simulink model "Gesamtmodell_Bahnplanung"  (R2015b)
settings: Solver=ode3  StartTime=0.0  StopTime=inf  FixedStep=dt  RelTol=1e-3
InitFcn:
  | Reglerauslegung
undefined symbols (not defined in the file): aMax, aMaxPsi, Blindzeit, Com1, dt, K1, K2, K3, Kx, Ky, none, sigbuilder_block, Tx, Ty, vMax, vMaxPsi
libraries: xpcrtudplib x11, simulink x6, xpcutilitieslib x4, xpcseriallib x1, slrtlib x1
(part 2 of 4)

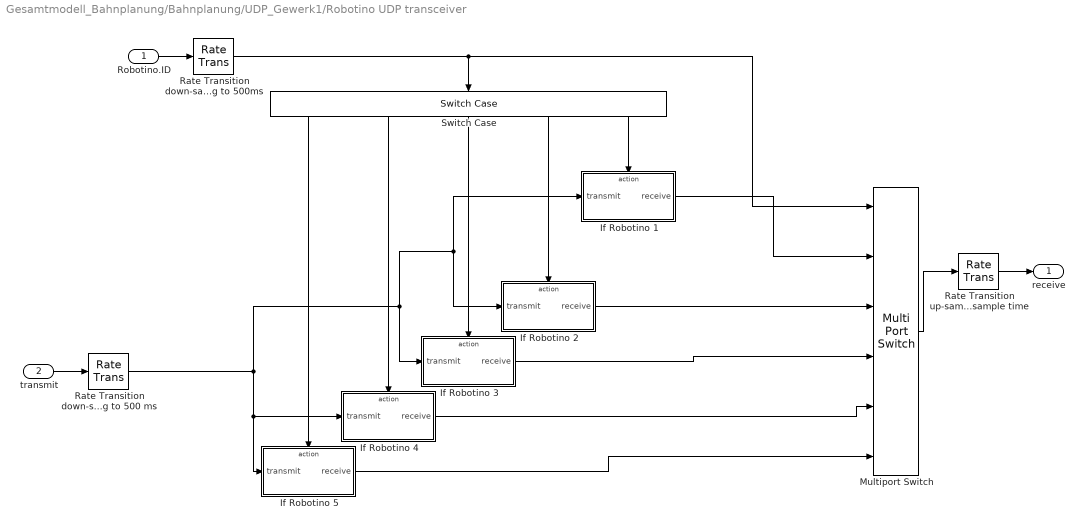
== system Gesamtmodell_Bahnplanung/Bahnplanung/UDP_Gewerk1/Robotino UDP transceiver ==
  Robotino.ID : Inport
  transmit : Inport  Port=2
  If Robotino 1 : Subsystem  TreatAsAtomicUnit=on
  If Robotino 2 : Subsystem  TreatAsAtomicUnit=on
  If Robotino 3 : Subsystem  TreatAsAtomicUnit=on
  If Robotino 4 : Subsystem  TreatAsAtomicUnit=on
  If Robotino 5 : Subsystem  TreatAsAtomicUnit=on
  Multiport Switch : MultiPortSwitch  Inputs=5
  Rate Transition down-sampling to 500 ms : RateTransition  OutPortSampleTime=0.5
  Rate Transition down-sampling to 500ms : RateTransition  OutPortSampleTime=0.5
  Rate Transition up-sampling to fundamental sample time : RateTransition
  Switch Case : SwitchCase  CaseConditions={5,4,3,2,1}  ShowDefaultCase=off
  receive : Outport
  wires:
  If Robotino 5/1(receive) -> Multiport Switch/6
  Switch Case/1 -> If Robotino 5/Action
  Rate Transition down-sampling to 500ms/1 -> Multiport Switch/1, Switch Case/1
  Robotino.ID/1 -> Rate Transition down-sampling to 500ms/1
  Rate Transition down-sampling to 500 ms/1 -> If Robotino 4/1(transmit), If Robotino 5/1(transmit), If Robotino 1/1(transmit), If Robotino 2/1(transmit), If Robotino 3/1(transmit)
  Rate Transition up-sampling to fundamental sample time/1 -> receive/1
  transmit/1 -> Rate Transition down-sampling to 500 ms/1
  If Robotino 4/1(receive) -> Multiport Switch/5
  If Robotino 2/1(receive) -> Multiport Switch/3
  If Robotino 3/1(receive) -> Multiport Switch/4
  If Robotino 1/1(receive) -> Multiport Switch/2
  Multiport Switch/1 -> Rate Transition up-sampling to fundamental sample time/1
  Switch Case/5 -> If Robotino 1/Action
  Switch Case/4 -> If Robotino 2/Action
  Switch Case/3 -> If Robotino 3/Action
  Switch Case/2 -> If Robotino 4/Action

== system Gesamtmodell_Bahnplanung/Regelung1/Receiver/UDP interface ==
  number of robot : Inport
  Receive : xpcrtudplib/UDP Receive  ipAddressVal=Use host-target connection  localPort=25000  rcvWidth=448  rcvFmAny=off  fmAddress=0.0.0.0  maxUDPQueue=8  sampleTime=-1
  Terminator : Terminator
  Unpack : xpcutilitieslib/Byte Unpacking   MaskUnpackedDataTypes={'double'}  MaskUnpackedDataSizes={[56]}  MaskAlignment=1
  stop signals : MATLAB Function  TreatAsAtomicUnit=on
  enable : Outport
  UDP data : Outport  Port=2
  wires:
  Unpack/1 -> stop signals/2(udp_in), UDP data/1
  Receive/1 -> Unpack/1
  Receive/2 -> Terminator/1
  stop signals/1(enable_out) -> enable/1
  number of robot/1 -> stop signals/1(rob_number)

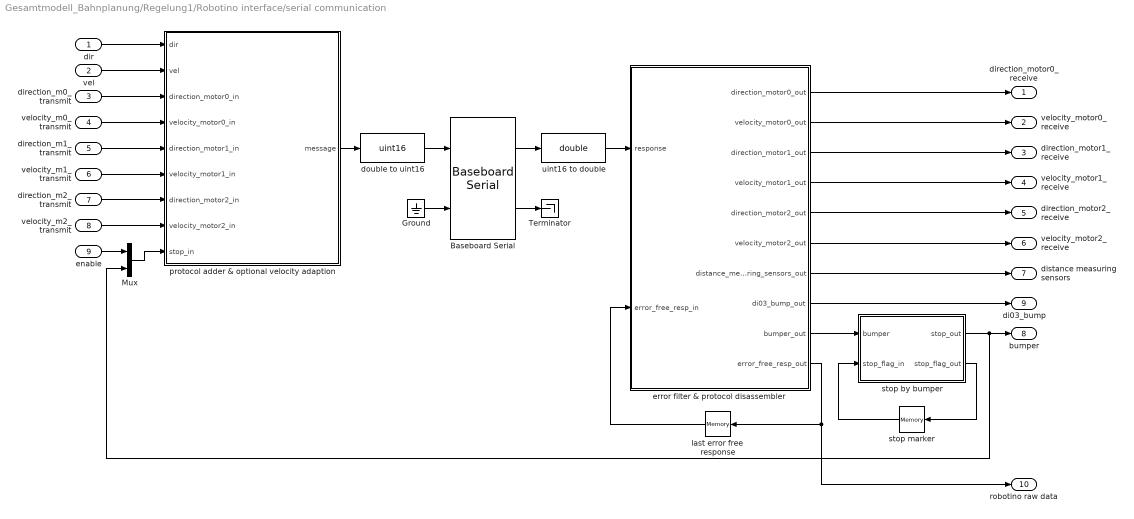
== system Gesamtmodell_Bahnplanung/Regelung1/Robotino interface/serial communication ==
  dir : Inport
  vel : Inport  Port=2
  direction_m0_transmit : Inport  Port=3
  velocity_m0_transmit : Inport  Port=4
  direction_m1_transmit : Inport  Port=5
  velocity_m1_transmit : Inport  Port=6
  direction_m2_transmit : Inport  Port=7
  velocity_m2_transmit : Inport  Port=8
  enable : Inport  Port=9
  Baseboard Serial : xpcseriallib/Mainboard/Baseboard Serial  group=Transmit Setup  port=2  irqnum=4  saddr1=0x3f8  saddr2=0x3e8  config=Com1/none  baud1=115200  parity1=None  ndata1=8  nstop1=1  fifomode1=16 deep  rlevel1=almost full  automode1=off  xmtfifosize1=10240  xmtdatatype1=count+16 bit uint  rcvfifosize1=10240  rcvmaxread1=101  rcvminread1=1  rcvusedelim1=on  rcvdelim1=99  rcvdatatype1=count+16 bit uint  rcvsampletime1=-1  baud2=115200  parity2=None  ndata2=8  nstop2=1  fifomode2=16 deep  rlevel2=almost full  automode2=off  xmtfifosize2=10240  xmtdatatype2=count+16 bit uint  rcvfifosize2=10240  rcvmaxread2=101  rcvminread2=1  rcvusedelim2=on  rcvdelim2=99  rcvdatatype2=count+16 bit uint  rcvsampletime2=-1
      link override FIFO read 1: maxsize=101  minsize=1  usedelimiter=on  delimiter=99  outputtype=count+16 bit uint  sampletime=dt / 2
      link override FIFO read 2: maxsize=101  minsize=1  usedelimiter=on  delimiter=99  outputtype=count+16 bit uint  sampletime=dt / 2
      link override FIFO write 1: size=1024  inputtype=count+16 bit uint  sampletime=-1  id=XMT channel 1, IRQ 4
      link override FIFO write 2: size=1024  inputtype=8 bit uint null terminated  id=XMT channel 2, IRQ 4
      link override Setup1: baud=115200  width=8  nstop=1  parity=None  fmode=16 deep  rlevel=half full  ctsmode=off
      link override Setup2: baud=4800  width=8  nstop=1  parity=None  fmode=16 deep  rlevel=half full  ctsmode=off
  Ground : Ground
  Mux : Mux  Inputs=2
  Terminator : Terminator
  double to uint16 : DataTypeConversion  OutDataTypeStr=uint16  RndMeth=Nearest
  error filter & protocol disassembler : MATLAB Function  TreatAsAtomicUnit=on
  last error free response : Memory  X0=[zeros(1,102)]
  protocol adder & optional velocity adaption : MATLAB Function  TreatAsAtomicUnit=on
  stop by bumper : MATLAB Function  TreatAsAtomicUnit=on
  stop marker : Memory  X0=[zeros(1,3)]
  uint16 to double : DataTypeConversion  OutDataTypeStr=double  RndMeth=Nearest
  direction_motor0_receive : Outport
  velocity_motor0_receive : Outport  Port=2
  direction_motor1_receive : Outport  Port=3
  velocity_motor1_receive : Outport  Port=4
  direction_motor2_receive : Outport  Port=5
  velocity_motor2_receive : Outport  Port=6
  distance measuring sensors : Outport  Port=7
  bumper : Outport  Port=8
  di03_bump : Outport  Port=9
  robotino raw data : Outport  Port=10
  wires:
  Ground/1 -> Baseboard Serial/2
  Baseboard Serial/2 -> Terminator/1
  double to uint16/1 -> Baseboard Serial/1
  protocol adder & optional velocity adaption/1(message) -> double to uint16/1
  stop marker/1 -> stop by bumper/2(stop_flag_in)
  stop by bumper/2(stop_flag_out) -> stop marker/1
  last error free response/1 -> error filter & protocol disassembler/2(error_free_resp_in)
  error filter & protocol disassembler/10(error_free_resp_out) -> last error free response/1, robotino raw data/1
  error filter & protocol disassembler/1(direction_motor0_out) -> direction_motor0_receive/1
  error filter & protocol disassembler/2(velocity_motor0_out) -> velocity_motor0_receive/1
  error filter & protocol disassembler/3(direction_motor1_out) -> direction_motor1_receive/1
  error filter & protocol disassembler/4(velocity_motor1_out) -> velocity_motor1_receive/1
  direction_m0_transmit/1 -> protocol adder & optional velocity adaption/3(direction_motor0_in)
  error filter & protocol disassembler/5(direction_motor2_out) -> direction_motor2_receive/1
  velocity_m0_transmit/1 -> protocol adder & optional velocity adaption/4(velocity_motor0_in)
  error filter & protocol disassembler/6(velocity_motor2_out) -> velocity_motor2_receive/1
  direction_m1_transmit/1 -> protocol adder & optional velocity adaption/5(direction_motor1_in)
  velocity_m1_transmit/1 -> protocol adder & optional velocity adaption/6(velocity_motor1_in)
  direction_m2_transmit/1 -> protocol adder & optional velocity adaption/7(direction_motor2_in)
  velocity_m2_transmit/1 -> protocol adder & optional velocity adaption/8(velocity_motor2_in)
  error filter & protocol disassembler/9(bumper_out) -> stop by bumper/1(bumper)
  stop by bumper/1(stop_out) -> bumper/1, Mux/2
  error filter & protocol disassembler/7(distance_measuring_sensors_out) -> distance measuring sensors/1
  Baseboard Serial/1 -> uint16 to double/1
  uint16 to double/1 -> error filter & protocol disassembler/1(response)
  enable/1 -> Mux/1
  dir/1 -> protocol adder & optional velocity adaption/1(dir)
  vel/1 -> protocol adder & optional velocity adaption/2(vel)
  Mux/1 -> protocol adder & optional velocity adaption/9(stop_in)
  error filter & protocol disassembler/8(di03_bump_out) -> di03_bump/1

== system Gesamtmodell_Bahnplanung/Regelung1/getRobotinoID/getIDfromFlash ==
  Trigger : TriggerPort
  From File : slrtlib/Target Management/From File   filename='robotino.id'  dataSize=8  bufSize=2000  readSize=512  EOFOption=Seek to beginning  sampTime=-1  show2ports=off
  Unpack : xpcutilitieslib/Byte Unpacking   MaskUnpackedDataTypes={'double'}  MaskUnpackedDataSizes={[1]}  MaskAlignment=1
  RobotinoID : Outport
  wires:
  From File/1 -> Unpack/1
  Unpack/1 -> RobotinoID/1

== system Gesamtmodell_Bahnplanung/Bahnplanung/UDP_Gewerk1/Robotino UDP transceiver/If Robotino 1 ==
  transmit : Inport
  Action Port : ActionPort  ActionType=case
  Receive from all : xpcrtudplib/UDP Receive  ipAddressVal=Use host-target connection  localPort=25011  rcvWidth=36  rcvFmAny=off  fmAddress=0.0.0.0  maxUDPQueue=8  sampleTime=-1
  Send to all : xpcrtudplib/UDP Send  ipAddressVal=Use host-target connection  localPort=-1  toAddress=255.255.255.255  toPort=25010  sampleTime=-1
  Terminator : Terminator
  receive : Outport
  wires:
  transmit/1 -> Send to all/1
  Receive from all/2 -> Terminator/1
  Receive from all/1 -> receive/1

== system Gesamtmodell_Bahnplanung/Bahnplanung/UDP_Gewerk1/Robotino UDP transceiver/If Robotino 2 ==
  transmit : Inport
  Action Port : ActionPort  ActionType=case
  Receive from all : xpcrtudplib/UDP Receive  ipAddressVal=Use host-target connection  localPort=25012  rcvWidth=36  rcvFmAny=off  fmAddress=0.0.0.0  maxUDPQueue=8  sampleTime=-1
  Send to all : xpcrtudplib/UDP Send  ipAddressVal=Use host-target connection  localPort=-1  toAddress=255.255.255.255  toPort=25020  sampleTime=-1
  Terminator : Terminator
  receive : Outport
  wires:
  transmit/1 -> Send to all/1
  Receive from all/2 -> Terminator/1
  Receive from all/1 -> receive/1

== system Gesamtmodell_Bahnplanung/Bahnplanung/UDP_Gewerk1/Robotino UDP transceiver/If Robotino 3 ==
  transmit : Inport
  Action Port : ActionPort  ActionType=case
  Receive from all : xpcrtudplib/UDP Receive  ipAddressVal=Use host-target connection  localPort=25013  rcvWidth=36  rcvFmAny=off  fmAddress=0.0.0.0  maxUDPQueue=8  sampleTime=-1
  Send to all : xpcrtudplib/UDP Send  ipAddressVal=Use host-target connection  localPort=-1  toAddress=255.255.255.255  toPort=25030  sampleTime=-1
  Terminator : Terminator
  receive : Outport
  wires:
  transmit/1 -> Send to all/1
  Receive from all/2 -> Terminator/1
  Receive from all/1 -> receive/1

== system Gesamtmodell_Bahnplanung/Bahnplanung/UDP_Gewerk1/Robotino UDP transceiver/If Robotino 4 ==
  transmit : Inport
  Action Port : ActionPort  ActionType=case
  Receive from all : xpcrtudplib/UDP Receive  ipAddressVal=Use host-target connection  localPort=25014  rcvWidth=36  rcvFmAny=off  fmAddress=0.0.0.0  maxUDPQueue=8  sampleTime=-1
  Send to all : xpcrtudplib/UDP Send  ipAddressVal=Use host-target connection  localPort=-1  toAddress=255.255.255.255  toPort=25040  sampleTime=-1
  Terminator : Terminator
  receive : Outport
  wires:
  transmit/1 -> Send to all/1
  Receive from all/2 -> Terminator/1
  Receive from all/1 -> receive/1

== system Gesamtmodell_Bahnplanung/Bahnplanung/UDP_Gewerk1/Robotino UDP transceiver/If Robotino 5 ==
  transmit : Inport
  Action Port : ActionPort  ActionType=case
  Receive from all : xpcrtudplib/UDP Receive  ipAddressVal=Use host-target connection  localPort=25015  rcvWidth=36  rcvFmAny=off  fmAddress=0.0.0.0  maxUDPQueue=8  sampleTime=-1
  Send to all : xpcrtudplib/UDP Send  ipAddressVal=Use host-target connection  localPort=-1  toAddress=255.255.255.255  toPort=25050  sampleTime=-1
  Terminator : Terminator
  receive : Outport
  wires:
  Receive from all/1 -> receive/1
  Receive from all/2 -> Terminator/1
  transmit/1 -> Send to all/1

== stateflow chart Gesamtmodell_Bahnplanung/Bahnplanung/Aufrag_steuern ==
  settings: updateMethod=DISCRETE  sampleTime=dt
  state Auftragskoordination
    state KeinWerkstueckAufgenommen
      entry:Werkstueck=0,
      AktuellesZiel=WerkstueckPos,
      Bearbeitet=1;
    state WerkstueckAbgelegt
      entry:Werkstueck=0,
      AktuellesZiel=ZielPos,
      Bearbeitet=1;
    state AufAuftragWarten
      entry:Werkstueck=0,
      AktuellesZiel=100
      Bearbeitet=0;
    state Laden
      entry:Werkstueck=0,
      AktuellesZiel=WerkstueckPos,
      Bearbeitet=1;
    state Ladenabgeschlossen
      entry:Werkstueck=0,
      AktuellesZiel=WerkstueckPos,
      Bearbeitet=1;
    state WerkstueckAufgenommen
      entry:Werkstueck=1,
      AktuellesZiel=ZielPos,
      Bearbeitet=1;
    (default) -> AufAuftragWarten
    KeinWerkstueckAufgenommen -> AufAuftragWarten [order 2] : [Fehler==1&& Transportbereich==1]
    WerkstueckAbgelegt -> AufAuftragWarten : [Werkstueckerkannt==0 && Transportbereich==1]
    AufAuftragWarten -> KeinWerkstueckAufgenommen [order 1] : [NeuerAuftrag ==1 && WerkstueckPos< 80 && Fehler==0]
    WerkstueckAufgenommen -> AufAuftragWarten [order 2] : [Fehler==2  && Transportbereich==1]
    AufAuftragWarten -> Laden [order 2] : [NeuerAuftrag ==1 && WerkstueckPos>= 80]
    Ladenabgeschlossen -> AufAuftragWarten : [Transportbereich==1]
    WerkstueckAufgenommen -> WerkstueckAbgelegt [order 3] : [Werkstueckerkannt==0 && Transportbereich==0]
    KeinWerkstueckAufgenommen -> WerkstueckAufgenommen [order 1] : [Werkstueckerkannt==1 && Transportbereich==1]
    Laden -> Ladenabgeschlossen : [Status==4]
    WerkstueckAufgenommen -> WerkstueckAufgenommen [order 1] : [Fehler==3]
  data: NeuerAuftrag input; WerkstueckPos input; ZielPos input; AktuellesZiel output; Werkstueck output; Werkstueckerkannt input; Transportbereich input; Bearbeitet output; Status input; Fehler input

== matlab function Gesamtmodell_Bahnplanung/Bahnplanung/Fehler_erkennen ==
  data: Fehler_IN input; Reset input; Transportbereich input; Werkstueckerkannt input; Werkstueck input; Fehler_OUT output; Fehler_alt input
function Fehler_OUT       = fcn(Fehler_IN ,Reset, Transportbereich, Werkstueckerkannt,Werkstueck, Fehler_alt)
if Reset == 1 || Fehler_IN ~= 0 %Reset des Fehlers
    Fehler_OUT=Fehler_IN;
else
    if Transportbereich == 1 && Werkstueckerkannt~=1 && Werkstueck == 1 %Werkstück während der Fahrt verloren erkennen
       Fehler_OUT = 2;
    else
       Fehler_OUT=Fehler_alt; 
    end 
end
end

== stateflow chart Gesamtmodell_Bahnplanung/Bahnplanung/Fifo_bestimmen/Fifo_Position_bestimmen ==
  settings: updateMethod=DISCRETE  sampleTime=dt
  state FIFOStationen
    state Auftrag_Roboter_1
    state Zielbereich_untersuchen
      entry:
      ersterFifo=floor(Zielstation/2)*3+2*mod(Zielstation,2)+1;
    state Fifo_einfachbesetzt1
      entry:
      zweiterFifo=floor(Zielstation/2)*3+1+1,
      Fifo=2;
    state Fifo_frei
      entry:
      Fifo=1;
    state Uebergabepunkt_gleich_Zielpunkt
      entry:
      Fifo=0;
    state Fifo_doppelt_besetzt
      entry:
      dritterFifo=floor(Zielstation/2)*3+2-2*mod(Zielstation,2)+1,
      Fifo=3;
    state Fifo_voll
      entry:
      Fifo=4;
    (default) -> Auftrag_Roboter_1
    Auftrag_Roboter_1 -> Zielbereich_untersuchen : [Zielposition>-1]
    Zielbereich_untersuchen -> Uebergabepunkt_gleich_Zielpunkt [order 2]
    Zielbereich_untersuchen -> Fifo_einfachbesetzt1 [order 1] : [(FifoArray(ersterFifo)~=0)| (FifoArray(ersterFifo)==0 & StationArray(Zielstation+1)~=0) ]
    Uebergabepunkt_gleich_Zielpunkt -> Zielbereich_untersuchen
    Fifo_einfachbesetzt1 -> Fifo_frei [order 2] : [FifoArray(ersterFifo)==0]
    Fifo_frei -> Uebergabepunkt_gleich_Zielpunkt : [ StationArray(Zielstation+1)==0]
    Fifo_einfachbesetzt1 -> Fifo_doppelt_besetzt [order 1] : [(FifoArray(zweiterFifo)~=0)]
    Fifo_doppelt_besetzt -> Fifo_einfachbesetzt1 [order 1] : [FifoArray(zweiterFifo)==0]
    Fifo_voll -> Fifo_doppelt_besetzt : [FifoArray(dritterFifo)==0]
    Fifo_doppelt_besetzt -> Fifo_voll [order 2] : [(FifoArray(dritterFifo)~=0)]
  state Wartebereich
    entry: Fifo=4;
  state Ladestation
    entry: Fifo=0;
  state Ladestation1
    entry: Fifo=4;
  FIFOStationen -> FIFOStationen [order 1] : [after(1000, tick)]
  (default) -> Wartebereich
  Wartebereich -> FIFOStationen [order 1] : [Zielstation<8]
  FIFOStationen -> Wartebereich [order 2] : [Zielstation==10]
  Ladestation -> Wartebereich [order 1] : [Zielstation==10]
  Wartebereich -> Ladestation [order 2] : [Zielstation>=8 & Zielstation<10]
  Ladestation -> FIFOStationen [order 2] : [Zielstation<8]
  FIFOStationen -> Ladestation [order 3] : [Zielstation>=8 & Zielstation<10]
  Ladestation -> Ladestation1 [order 3] : [Ladenarray(1)~=0]
  Ladestation1 -> Ladestation : [Ladenarray(1)==0]
  data: FifoArray input; Zielposition input; Zielstation input; Fifo output; StationArray input; dritterFifo local; zweiterFifo local; ersterFifo local; Ladenarray input

== matlab function Gesamtmodell_Bahnplanung/Bahnplanung/Fifo_bestimmen/Fifo_Merker_bestimmen ==
  data: StationArray1 output; Robbi input; FifoArray input; FifoArray1 output; LadeArray1 output; LadeArray input
function [StationArray1,FifoArray1,LadeArray1]= fcn(Robbi,FifoArray,LadeArray)
X=zeros([1 4]);
Y=zeros([1 4]);
X=[Robbi(1) Robbi(4) Robbi(7) Robbi(10)];
Y=[Robbi(2) Robbi(5) Robbi(8) Robbi(11)];
FifoArray1=zeros([1 12]);
FifoArray1=FifoArray(1:12);
StationArray1=zeros([1 8]);
LadeArray1=zeros([1 2]);
LadeArray1=LadeArray(1:2);
N=zeros([1 4]);
S=zeros([1 4]);
L=zeros([1 4]);
  for n= 1 : 1 : 4
    L(n)=round((Y(n)-2592)/500)+1; % Berechnung in welcher Ladestation sich der Robotino befindet
    N(n)=round((X(n)-703)/425)+1;  % Berechnung in welchem Fifo der Roboter sich befindet
    S(n)=round((X(n)-900)/560)+1;  % Berechnung in welcher Station der Roboter sich befindet
     if (X(n)<=6000 || X(n)>6500)  % Ladearray zurücksetzten
        for i=1:2
            if LadeArray1(i)==n
                LadeArray1(i)=0;
            end
        end
     end
    if (X(n)>6000 && X(n)<=6500 && Y(n)>2300 && Y(n)<=3300 && L(n)<=2 && L(n)>0)%Ladearray setzten wenn ein Robotino drin steht
        LadeArray1(1)=n;
        LadeArray1(2)=n;
    end  
   
    for i=1:8 % Stationsarray zurücksetzten
          if StationArray1(i)==n
                StationArray1(i)=0;
          end
    end
    if (Y(n)>2450 && Y(n)<3300 && X(n)<5100 && S(n)<=8 && S(n)>0) %% Setzen des Stationsarray gleiczeitig rücksetzten des ersten fifos
         for i=1:12
            if FifoArray1(i)==n
                FifoArray1(i)=0;
            end
         end
       
        StationArray1(S(n))=n;
    end
    if (Y(n)<450 && X(n)>100 && X(n)<6000 && N(n)<=12 && N(n)>0) % Setzten der aktuellen Fifoposition
        for i=1:12
            if FifoArray1(i)==n
                FifoArray1(i)=0;
            end
        end
            FifoArray1(N(n))=n;
    end  
    if (X(n)>6000 && Y(n)<2000)% Rücksetzen der FIFOs auf Warteposition
        for i=1:12
            if FifoArray1(i)==n
                FifoArray1(i)=0;
            end
        end
    end
  end
end

== matlab function Gesamtmodell_Bahnplanung/Bahnplanung/Fifo_bestimmen/Zielkoordinaten_bestimmen ==
  data: Fifo input; Zielstation input; Endposition output; RoboterID input
function Endposition = fcn(Fifo,Zielstation,RoboterID)
Endposition=zeros([1 2]);

WartepositionX= [6200 6800 7200 7350 7200]; % Wartepositionen X koordinate
WartepositionY= [100 175 550 1150 1750];    % Wartepositionen Y koordinate

% Übergabepositionen der Stationen
StationvorneX=[853 1361 2058 2559 3256 3762 4448 4953 5965 5965];
StationvorneY=[2300 2300 2300 2300 2300 2300 2300 2300 3080 2593];

% Fifoposition bestimmen
ersterFifo=floor(Zielstation/2)*3+2*mod(Zielstation,2);
zweiterFifo=floor(Zielstation/2)*3+1;
dritterFifo=floor(Zielstation/2)*3+2-2*mod(Zielstation,2);

if Fifo==0 %Übergabepunkt als Ziel übernehmen
    Endposition(1)=StationvorneX(Zielstation+1);
    Endposition(2)=StationvorneY(Zielstation+1);
    %Fifopositionen als Ziel übernehmen
    else if Fifo==1 
        Endposition(1)= ersterFifo*425+703;
        Endposition(2)= 250;
       
    else if Fifo==2
            Endposition(1)= zweiterFifo*425+703;
            Endposition(2)= 250;
        
    else if Fifo==3
            Endposition(1)= dritterFifo*425+703;
            Endposition(2)= 250;
            else
            Endposition(2)= WartepositionY(RoboterID);
            Endposition(1)= WartepositionX(RoboterID);
        end
        end
        end
end
end

== matlab function Gesamtmodell_Bahnplanung/Bahnplanung/Fifo_bestimmen/Zielfach_formatieren ==
  data: AktuellesZiel input; ZielPos output; Zielstation output
function [ZielPos,Zielstation]= fcn(AktuellesZiel)
ZielPos=mod(AktuellesZiel,10);
Zielstation=round(AktuellesZiel/10);

== matlab function Gesamtmodell_Bahnplanung/Bahnplanung/Fifo_bestimmen/Abstand_zum_Ziel_prüfen ==
  data: Erreicht output; AktuellePos input; Zielpos input
function Erreicht = fcn(AktuellePos,Zielpos)
Abstand=sqrt((AktuellePos(1)-Zielpos(1))^2+(AktuellePos(2)-Zielpos(2))^2);
if AktuellePos(2) >2000 && Abstand < 150 % Ziel erreicht wenn Abstand zum Ziel < 15 cm
    Erreicht=1;
else
    Erreicht=0;
end
end

== stateflow chart Gesamtmodell_Bahnplanung/Bahnplanung/Fahrmodus_steuern ==
  settings: updateMethod=DISCRETE  sampleTime=dt
  state KommunikationGW3
    state Fertigungsbereich
      entry:Transportbereich=0,
      Fertigungsbereich=1;
      state RFID_einchecken
        entry:Zielposition=Ziel-mod(Ziel,10)+3,
        Aktion_an_Position=Aktion_Warten,
        Status=2;
      state Startpunkt
        entry: Zielposition=Ziel-mod(Ziel,10);
        Aktion_an_Position=Aktion_Warten,
        Status=1;
      state Warten
        during: Bereich_Verlassen=1,
      state Warten1
      state Bereich_verlassen_hinten
        entry:Zielposition=Ziel-mod(Ziel,10)+4,
        Aktion_an_Position=Aktion_Warten,
        Status=1;
      state Bereich_verlassen_vorne1
        entry:Zielposition=Ziel-mod(Ziel,10),
        Aktion_an_Position=Aktion_Warten,
        Status=1;
      state Position_anfahren
        entry:Zielposition=Ziel,
        Status=1,
        if Werkstueck==0
        Aktion_an_Position=Aktion_Aufnehmen;
        else
        Aktion_an_Position=Aktion_Ablegen;
        end
      state Bereich_verlassen
        entry:
        ersterFifo=floor(floor(Ziel/10)/2)*3+2*mod(floor(Ziel/10),2)+1;
        Aktion_an_Position=Aktion_Warten,
      state Warten2
      state RFID_auschecken
        entry:Zielposition=Ziel-mod(Ziel,10)+3,
        Aktion_an_Position=Aktion_Warten,
        Status=3;
      Startpunkt -> Startpunkt [order 1] : [Fehler==3]
      (default) -> Startpunkt
      Startpunkt -> RFID_einchecken [order 2] : [Ziel_anfordern==1 & Werkstueck==1]
      Startpunkt -> Position_anfahren [order 3] : [Ziel_anfordern==1 & Werkstueck==0]
      Position_anfahren -> Startpunkt [order 2] : [Fehler==3 & Ziel_anfordern==1]
      RFID_einchecken -> Warten1 : [Ziel_anfordern==1 ]
      Bereich_verlassen_hinten -> Warten : [Ziel_anfordern==1]
      Bereich_verlassen_vorne1 -> Warten : [Ziel_anfordern==1]
      Warten1 -> Position_anfahren : [RFID_Anmeldung==1]
      Bereich_verlassen -> Bereich_verlassen_hinten [order 2]
      Bereich_verlassen -> Bereich_verlassen_vorne1 [order 1] : [FifoArray(ersterFifo)==0]
      Position_anfahren -> Bereich_verlassen [order 1] : [Fehler==1 & Ziel_anfordern==1]
      Position_anfahren -> Bereich_verlassen [order 4] : [Ziel_anfordern==1 & (Aktion_an_Position==Aktion_Ablegen)]
      Position_anfahren -> RFID_auschecken [order 3] : [Ziel_anfordern==1 & (Aktion_an_Position==Aktion_Aufnehmen) & Fehler==0]
      Warten2 -> Bereich_verlassen : [RFID_Abmeldung==1]
      RFID_auschecken -> Warten2 : [Ziel_anfordern==1]
    state Transportbereich
      entry:Transportbereich=1,
      Zielposition=999,
      Fertigungsbereich=0,
      Bereich_Verlassen=0,
      Geladen=0,
      Status=1;
    state Ladestationanfahren2
      entry: Zielposition=100,
      Transportbereich=0,
      Fertigungsbereich=1,
      Status=1;
    state Warten3
    state Laden4
      entry: Zielposition=110,
      Transportbereich=0,
      Fertigungsbereich=1,
      Geladen=1,
      Status=4;
    state Laden2
      entry: Zielposition=110,
      Transportbereich=0,
      Fertigungsbereich=1,
      Status=1;
    state Ladestationanfahren1
      entry: Zielposition=80,
      Transportbereich=0,
      Fertigungsbereich=1,
      Status=1;
    state Laden3
      entry: Zielposition=90,
      Transportbereich=0,
      Fertigungsbereich=1,
      Geladen =1,
      Status=4;
    state Laden1
      entry: Zielposition=90,
      Transportbereich=0,
      Fertigungsbereich=1,
      Status=1;
    (default) -> Transportbereich
    Transportbereich -> Fertigungsbereich [order 1] : [(ZielStation_Erreicht==1) & (floor(Ziel/10)<=7)]
    Ladestationanfahren2 -> Transportbereich [order 2] : [ Geladen==1 & Ziel_anfordern==1 ]
    Fertigungsbereich -> Warten3 : [Bereich_Verlassen==1]
    Warten3 -> Transportbereich
    Transportbereich -> Ladestationanfahren2 [order 3] : [(ZielStation_Erreicht==1) & (floor(Ziel/10)==9)]
    Ladestationanfahren2 -> Laden2 [order 1] : [ Geladen==0 & Ziel_anfordern==1 ]
    Laden4 -> Ladestationanfahren2 : [Ladenabgeschlossen==1 ]
    Transportbereich -> Ladestationanfahren1 [order 2] : [(ZielStation_Erreicht==1) & (floor(Ziel/10)==8)]
    Ladestationanfahren1 -> Transportbereich [order 2] : [ Geladen==1 & Ziel_anfordern==1 ]
    Laden2 -> Laden4 : [Ziel_anfordern==1 ]
    Ladestationanfahren1 -> Laden1 [order 1] : [ Geladen==0 & Ziel_anfordern==1 ]
    Laden3 -> Ladestationanfahren1 : [Ladenabgeschlossen==1 ]
    Laden1 -> Laden3 : [Ziel_anfordern==1 ]
  data: Transportbereich output; Fertigungsbereich output; Ziel input; Zielposition output; Aktion_an_Position output double; Aktion_Warten local double =0; Aktion_Aufnehmen local double =1; Aktion_Ablegen local double =2; Werkstueck input double; Bereich_Verlassen local; Status output; FifoArray input; ersterFifo local double; Ziel_anfordern input; ZielStation_Erreicht input double; RFID_Anmeldung input; RFID_Abmeldung input; Ladenabgeschlossen input; Geladen local; Fehler input

== matlab function Gesamtmodell_Bahnplanung/Bahnplanung/Positionen_der_Robotinos_bestimmen ==
  data: UDPDaten input; RobPos output; RobotinoID input; StoerPos output size=[1 15]; altePos input size=[1 15]; altePos1 output size=[1 15]
function [RobPos,StoerPos,altePos1]      = fcn(UDPDaten , RobotinoID, altePos)
StoerPos=zeros([1 15]);
RobPos=zeros([1 3]);
altePos1=zeros([1 15]);
for x=0:4
    temp=abs(UDPDaten((x*3)+1:(x*3)+3));
    test=sum(temp);
    if(test==0) %Wenn die Position der Robotinos ~=[0 0 0] => keine Kameradaten
     altePos1((x*3)+1:(x*3)+3)=altePos((x*3)+1:(x*3)+3); 
    else
     altePos1((x*3)+1:(x*3)+3)=UDPDaten((x*3)+1:(x*3)+3);
    end
end
% Je nach Robotino Kameradaten auswählen
if RobotinoID==5
        RobPos(1:3) = altePos1(13:15);
        StoerPos(1:12)=altePos1(1:12);
    elseif RobotinoID == 4
        RobPos(1:3) = altePos1(10:12);
        StoerPos(1:9)=altePos1(1:9);
        StoerPos(10:12)=altePos1(13:15);
    elseif RobotinoID == 3
        RobPos(1:3) = altePos1(7:9);
        StoerPos(1:6)=altePos1(1:6);
        StoerPos(7:9)=altePos1(10:12);
        StoerPos(10:12)=altePos1(13:15);
    elseif RobotinoID == 2
        RobPos(1:3) = altePos1(4:6);
        StoerPos(1:3)=altePos1(1:3);
        StoerPos(4:9)=altePos1(7:12);
        StoerPos(10:12)=altePos1(13:15);
    elseif RobotinoID == 1
        RobPos(1:3) = altePos1(1:3);
        StoerPos(1:9)=altePos1(4:12);
        StoerPos(10:12)=altePos1(13:15);
        
end

== matlab function Gesamtmodell_Bahnplanung/Bahnplanung/Status_bestimmen ==
  data: Fehler_IN input; Status_IN input; Status output
function Status       = fcn(Fehler_IN ,Status_IN)
if Fehler_IN > 0 %Wenn Fehler aufgetreten Status anpassen
    Status = Fehler_IN + 4;
else
    Status = Status_IN;
end
end

== matlab function Gesamtmodell_Bahnplanung/Bahnplanung/Geschwindigkeit_transformieren ==
  data: Vektor input; V_RobX output; Winkel input; V_RobY output
function [V_RobX, V_RobY]= fcn(Vektor,Winkel)
% Globalen Geschwindigkeitsvektor in lokalen Geschwindigkeitsvektor
% umrechnen
V_RobX=(cos(Winkel)*Vektor(1)+sin(Winkel)*Vektor(2));
V_RobY=(cos(Winkel)*Vektor(2)-sin(Winkel)*Vektor(1));

== matlab function Gesamtmodell_Bahnplanung/Bahnplanung/UDP_Gewerk1/Winkelumrechnen ==
  data: RobWinkel input; Winkel output
function Winkel = fcn(RobWinkel)
Winkel=mod((RobWinkel*180/pi),360);
end

== matlab function Gesamtmodell_Bahnplanung/Bahnplanung/Geschwindigkeit_bestimmen/Ausweichmanöver_addieren ==
  data: Zone input; ZielPos input; RobotinoPos input; Ausweichwert input; Vektor_In input; Vektor output
function Vektor  = fcn(Zone,ZielPos,RobotinoPos,Ausweichwert,Vektor_In)
Vektor=zeros([1 2]);
%Ausweichmanöver
Distanz=sqrt((RobotinoPos(1)-ZielPos(1))^2+(RobotinoPos(2)-ZielPos(2))^2);
K=2;%neuer TEst letzter wert 1.4 2.5.18
AVX=zeros([1 4]);
AVY=zeros([1 4]);
 for x=1:4
 AVX(x)=-K*Ausweichwert(2,x)*cos(Ausweichwert(1,x));
 AVY(x)=-K*Ausweichwert(2,x)*sin(Ausweichwert(1,x));
 end
if (Zone==0) && ((Distanz > 300)&&(RobotinoPos(2)> 500)&&(RobotinoPos(1)> 500)&&(RobotinoPos(2)< 3000)&&(RobotinoPos(1)< 5000))
    if (RobotinoPos(2)> 2000)&& Vektor(1)<=0
        VektorX=Vektor_In(1);
        VektorY=Vektor_In(2);
    else
        VektorX=Vektor_In(1)+sum(AVX);
        VektorY=Vektor_In(2)+sum(AVY);
    end
else
 VektorX=Vektor_In(1);
 VektorY=Vektor_In(2);
end

%Bremsen vor dem Ziel

MaxDis=1000;
if Distanz > MaxDis
Vektor(1) = VektorX;
Vektor(2) = VektorY;
else
Vektor(1) = VektorX*Distanz/MaxDis;
Vektor(2) = VektorY*Distanz/MaxDis;  
end

end

== matlab function Gesamtmodell_Bahnplanung/Bahnplanung/Geschwindigkeit_bestimmen/Ausweichrichtung_bestimmen ==
  data: RobotinoPos input; StoerPos input; Vektor input; Ausweich output
function Ausweich  = fcn(RobotinoPos, StoerPos, Vektor)
Abstand=zeros([2 4]);
Ausweich=zeros([2 4]);%Zeile1 =Richtung(winkel in Rad) Zeile2=Intensität
for i=1:4
    %Abstand der Robotinos bestimmen
    Abstand(1,i)=-RobotinoPos(1)+StoerPos(1+((i-1)*3));
    Abstand(2,i)=-RobotinoPos(2)+StoerPos(2+((i-1)*3));
    Hyp=sqrt(Abstand(1,i)^2+Abstand(2,i)^2);
    if(Hyp==0)
        Hyp=1e-22;
    end
    if Hyp <=1000 %Wenn Robotino näher als ein Meter Ausweichrichtung bestimmen
        if Abstand(1,i) >= 0
             Ausweich(1,i)=+asin(Abstand(2,i)/Hyp)-pi/2;
        else
            Ausweich(1,i)=-asin(Abstand(2,i)/Hyp)+pi/2;
        end
        %Fahrtrichtung bestimmen
        HypZiel=sqrt(Vektor(1)^2+Vektor(2)^2);
         if Vektor(1) >= 0
            Fahrwinkel=+asin(Vektor(2)/HypZiel);
        else
            Fahrwinkel=-asin(Vektor(2)/HypZiel)+pi;
        end
        if abs(Fahrwinkel-(Ausweich(1,i)+pi/2))<=pi %Wenn Fahrtrichtung = Robotinorichtung +- pi/6 Toleranz
            if((Fahrwinkel-(Ausweich(1,i)+pi/2)) <= pi/6) && ((Fahrwinkel-(Ausweich(1,i)+pi/2))  >= -pi/6)
            Ausweich(2,i)=1;
             else
           Ausweich(2,i)=0; 
            end
        else
            if((2*pi)-abs(Fahrwinkel-(Ausweich(1,i)+pi/2)) <= pi/6) 
            Ausweich(2,i)=1;
             else
           Ausweich(2,i)=0; 
            end
        end
    else
        Ausweich(1,i)=0;
        Ausweich(2,i)=0;
    end
    % Wenn die Robotinos im FiFo stehet kein Ausweichmanöver ausführen
    if StoerPos(2+((i-1)*3))<300
        Ausweich(2,i)=0;
    end
end

== matlab function Gesamtmodell_Bahnplanung/Bahnplanung/Geschwindigkeit_bestimmen/Fahrende_Robotinos_erkennen ==
  data: Stoerpos input; Robotinofaehrt output; Stoeralt input
function Robotinofaehrt = fcn(Stoerpos,Stoeralt)
Robotinofaehrt=zeros([1 4]);
for x=1:4 % Wenn Robotinos mehr als 10mm/s zurückgelegt hat wird er als fahrend betrachtet
    if (abs(Stoeralt(1+(3*(x-1)))-Stoerpos(1+(3*(x-1)))) >= 10) && (abs(Stoeralt(2+(3*(x-1)))-Stoerpos(2+(3*(x-1)))) >= 10)
        Robotinofaehrt(x)=1;
    else
        Robotinofaehrt(x)=0;
    end
end

== stateflow chart Gesamtmodell_Bahnplanung/Regelung1/Zustandsautomat/FertigunsbereichsLogik1 ==
  state Greifer [parallel]
    settings: executionOrder=2
    state GreiferAuf
      entry: GreiferPose=0;
    state GreiferZu
      entry: GreiferPose=1;
    (default) -> GreiferAuf : [LSG == 0]
    GreiferAuf -> GreiferZu : [GreiferPose == 1]
    GreiferZu -> GreiferAuf : [LSG==0 || GreiferPose ==0]
  state Hauptding [parallel]
    settings: executionOrder=1
    state Warten
      entry: ZielAnfordern = 1;
      exit: ZielAnfordern = 0,
      FehlerNr = 0;
    state Neues_Ziel_erhalten
    state StationNichtErreich
      entry: FehlerNr = 3,
      korrektur = 0;
    state KeinWSgefunden
      entry: FehlerNr = 1,
    state Vorposition_vor_FachAnfahrt
      entry: StationsNr = Ziel + 5;
    state Vorposition_nach_FachAnfahrt
      entry: StationsNr = letztesZiel + 5;
    state Ziel_anfahren
      entry: StationsNr = Ziel;
    state Losfahren
      entry: enable = 1,
      Neue_Planung = 1;
      exit: Neue_Planung = 0;
    note: Warten<=
    state Loslassen
      entry: GreiferPose = 0;
    state Greifen
      entry: GreiferPose = 1;
    state FachAnfahren
    state SonstigePositionAnfahren
    state Station_erreicht
      entry: enable = 0,
      exit: letztesZiel = StationsNr;
    (default) -> Warten
    Warten -> Warten [order 1] : [Ziel == 999]/{letztesZiel = 999}
    Warten -> Neues_Ziel_erhalten [order 2] : [Ziel ~= letztesZiel]
    StationNichtErreich -> Warten
    KeinWSgefunden -> Warten
    Greifen -> Warten [order 2]
    Loslassen -> Warten
    Station_erreicht -> Warten [order 5]
    Neues_Ziel_erhalten -> Vorposition_vor_FachAnfahrt [order 2] : [istEinFach(Ziel) &&  ...
        |  ~istVorpositionDesFachs(Ziel, letztesZiel)]
    Neues_Ziel_erhalten -> Vorposition_nach_FachAnfahrt [order 1] : [istEinFach(letztesZiel)]
    Neues_Ziel_erhalten -> Ziel_anfahren [order 3]
    Station_erreicht -> Neues_Ziel_erhalten [order 2] : [StationsNr ~= Ziel]
    Station_erreicht -> StationNichtErreich [order 1] : [korrektur >= 2]
    Greifen -> KeinWSgefunden [order 1] : [LSG == 0]
    Ziel_anfahren -> Losfahren
    Vorposition_nach_FachAnfahrt -> Losfahren
    FachAnfahren -> Vorposition_vor_FachAnfahrt [order 1] : [korrektur >= 2]
    FachAnfahren -> Vorposition_vor_FachAnfahrt [order 2] : [after(2.5/dt, tick)]
        | /{korrektur = korrektur+1;}
    Vorposition_vor_FachAnfahrt -> Losfahren
    Losfahren -> FachAnfahren [order 1] : [istEinFach(StationsNr)]
    Losfahren -> SonstigePositionAnfahren [order 2] : [~istEinFach(StationsNr)]
    Station_erreicht -> Loslassen [order 4] : [AktionAnZiel == 2]
    Station_erreicht -> Greifen [order 3] : [AktionAnZiel == 1]
    FachAnfahren -> Station_erreicht [order 3] : [TasterGreifer]
        | /{korrektur = 0}
    SonstigePositionAnfahren -> Station_erreicht : [zielPositionErreicht]
  data: Ziel function_input double; letztesZiel function_input double; antwort function_output double; ziel function_input double; antwort function_output double; Ziel input double; AktionAnZiel input double; ZielAnfordern output double =0; letztesZiel local double =0; enable output double =0; GreiferPose output double; zielPositionErreicht input; StationsNr output double =0; korrektur output double =0; Neue_Planung output double; LSG input double; TasterGreifer input double; dt parameter; FehlerNr output double; Versuch local double =0; counter local double
  function antwort = istVorpositionDesFachs(Ziel, letztesZiel):
    | function antwort = istVorpositionDesFachs(Ziel, letztesZiel)
    | 
    |     if (letztesZiel - 5) == Ziel
    |         % Fachnummer + 5 = Nummer der Vorposition
    |         antwort = 1;
    |     else
    |         antwort = 0;
    |     end
    | 
    | end
  function antwort = istEinFach(ziel):
    | function antwort = istEinFach(ziel)
    |  
    |     if 0 < mod(ziel, 10) &&  mod(ziel, 10) < 4
    |         antwort = 1;
    |     else
    |         antwort = 0;
    |     end
    | 
    | end

== matlab function Gesamtmodell_Bahnplanung/Regelung1/Kalman1 ==
  data: vxZustand input; vyZustand input; vPsiZustand input; PsiZustand input; xZustand input; yZustand input; enable input; dt parameter; vx output; vy output; vpsi output; pospsi output; posx output; posy output; enableBeob output; Blindzeit parameter
function [vx,vy,vpsi,pospsi,posx,posy,enableBeob] = fcn(vxZustand,vyZustand,vPsiZustand,PsiZustand,xZustand,yZustand,enable,dt,Blindzeit)

persistent A H Q RPosX RPosY RPosPsi 
persistent x P
persistent firstRun found counter
QVelX = 0.01;
QVelY = 0.01;
QVelPsi = 0.01;
QPosX = 0.01;
QPosY = 0.01;
QPosPsi = 0.1;



if isempty(firstRun)
found = 0;
x = [0; 0; 0; 0; 2000; 1600];
    

A= [1       0       0       0       0       0;
    0       1       0       0       0       0;
    0       0       1       0       0       0;
    0       0       dt      1       0       0;
    dt      0       0       0       1       0;
    0       dt      0       0       0       1];
    
H = [0 0 0 1 0 0;
     0 0 0 0 1 0;
     0 0 0 0 0 1];

Q = [QVelX       0       0       0       0       0;
     0       QVelY       0       0       0       0;
     0          0       QVelPsi    0       0       0;
     0          0       0       QPosX    0       0;
     0          0       0       0       QPosY    0;
     0          0       0       0       0    QPosPsi];
   
  RPosX = 0.340050836575258;
  RPosY =0.684587581598845;
  RPosPsi=5.754253525875726e-05;

  P =  [1       0       0       0       0       0;
        0       1       0       0       0       0;
        0       0       1       0       0       0;
        0       0       0       1000       0       0;
        0       0       0       0       1000       0;
        0       0       0       0       0       1000];
  
  firstRun = 1; 
  counter = 0;
end
%Prediction
x =[vxZustand ; vyZustand; vPsiZustand;x(4:end,1)];

x = A*x;  
P = A*P*A' + Q;  
counter = counter+1;
dist=0;
Rnow=[RPosX 0 0; 0 RPosY 0; 0 0 RPosPsi];


%Correction
if enable == 1
    z = [PsiZustand;xZustand;yZustand];
    % Reduzierung der Glaubwürdigkeit bei weit entfernten Messungen
    dist = sqrt(abs(z(2)-x(5))^2 + abs(z(3)-x(6))^2);
    counter =0;
    
    if dist > 20
        found = 1;
    end
    K =    P*H'*inv(H*P*H' + Rnow); 
    x = x + K*(z - H*x);
    P = P - K*H*P;
end

if counter>= (Blindzeit/dt)
    found = 0;
end
enableBeob = found;

vx      = x(1);
vy      = x(2);
vpsi    = x(3);
pospsi  = x(4);
posx    = x(5);
posy    = x(6);

== matlab function Gesamtmodell_Bahnplanung/Bahnplanung/Geschwindigkeit_bestimmen/IR_Daten_Erfassen ==
  data: RobotinoDaten input; IRWerte output; RobPos input
function IRWerte = fcn(RobotinoDaten,RobPos)
IRWerte=zeros([2 9]);
IRDaten=zeros([1 9]);
IRDaten=RobotinoDaten(6:14);

for x=1:9 %IR Hindernispositionen in globalen Koordinaten bestimmen
    if  (isnan(IRDaten(x))==0) && (IRDaten(x) <= 150)
    IRWerte(1,x)=cos(((x-1)*40*pi/180)+RobPos(3))*(IRDaten(x)+200)+RobPos(1);
    IRWerte(2,x)=sin(((x-1)*40*pi/180)+RobPos(3))*(IRDaten(x)+200)+RobPos(2);
    else
    IRWerte(1,x)=NaN;
    IRWerte(2,x)=NaN;
    end
end

== matlab function Gesamtmodell_Bahnplanung/Bahnplanung/Geschwindigkeit_bestimmen/Geschwindigkeitsvektor_bestimmen ==
  data: StoerPos input; IRWerte input; RobotinoPos input; RobotinoFaehrt input; ZielPos input; Vektor output; Zone output; AlteZone input; FifoArray input
function [Vektor,Zone] = fcn( StoerPos, IRWerte,RobotinoPos,RobotinoFaehrt,ZielPos,AlteZone,FifoArray)
% Stationspositionen
Stationen=[1103,2308,3507,4694,6300,6300; 
            2832,2832,2832,2832,2608,3085;];
Vektor=zeros([1 2]);
% Stationen Einflussvektor
K=500;
sigma=187;
SVX=zeros([1 6]);
SVY=zeros([1 6]);
for x=1:4 % Stationspotentiale
SVX(x)= -K*exp(-((RobotinoPos(1)-Stationen(1,x))^2+(RobotinoPos(2)-Stationen(2,x))^2)/(2*(sigma^2)))*((RobotinoPos(1)-Stationen(1,x))/(sigma^2));
SVY(x)= -K*exp(-((RobotinoPos(1)-Stationen(1,x))^2+(RobotinoPos(2)-Stationen(2,x))^2)/(2*(sigma^2)))*((RobotinoPos(2)-Stationen(2,x))/(sigma^2));
end
K=300;
sigma=100; 
for x=5:6 % Ladestation
SVX(x)= -K*exp(-((RobotinoPos(1)-Stationen(1,x))^2+(RobotinoPos(2)-Stationen(2,x))^2)/(2*(sigma^2)))*((RobotinoPos(1)-Stationen(1,x))/(sigma^2));
SVY(x)= -K*exp(-((RobotinoPos(1)-Stationen(1,x))^2+(RobotinoPos(2)-Stationen(2,x))^2)/(2*(sigma^2)))*((RobotinoPos(2)-Stationen(2,x))/(sigma^2));
end
% Zielvektor
K=0.7;%=0.5;
if (RobotinoPos(1)~=ZielPos(1)) && (RobotinoPos(2)~=ZielPos(2))  
    ZVX = K*(RobotinoPos(1)-ZielPos(1))/sqrt((RobotinoPos(1)-ZielPos(1))^2 +(RobotinoPos(2)-ZielPos(2))^2);
    ZVY = K*(RobotinoPos(2)-ZielPos(2))/sqrt((RobotinoPos(1)-ZielPos(1))^2 +(RobotinoPos(2)-ZielPos(2))^2);
else
    ZVX=0;
    ZVY=0;
end

%Robtino Stoervektoren
RVX=zeros([1 4]);
RVY=zeros([1 4]);
for x=1:4
if (RobotinoFaehrt(x) == 1) && (RobotinoPos(2)> 500)
K=1300;
sigma=240;
elseif (RobotinoPos(2)> 2500)
K=700;
sigma=200;
elseif (RobotinoPos(2)< 2500)
K=1000;
sigma=200;
end
RVX(x)=-K*exp(-((RobotinoPos(1)-StoerPos((x*3)-2))^2+(RobotinoPos(2)-StoerPos((x*3)-1))^2)/(2*(sigma^2)))*((RobotinoPos(1)-StoerPos((x*3)-2))/(sigma^2));
RVY(x)=-K*exp(-((RobotinoPos(1)-StoerPos((x*3)-2))^2+(RobotinoPos(2)-StoerPos((x*3)-1))^2)/(2*(sigma^2)))*((RobotinoPos(2)-StoerPos((x*3)-1))/(sigma^2));
end

%Infrarot Einflussvektor
K=600;
sigma=250;
IRVX=zeros([1 9]);
IRVY=zeros([1 9]);
for x=1:9
    if(isnan(IRWerte(1,x))==0)||(isnan(IRWerte(2,x))==0)
       if (RobotinoPos(2)> 500)
    IRVX(x)=-K*exp(-((RobotinoPos(1)-IRWerte(1,x))^2+(RobotinoPos(2)-IRWerte(2,x))^2)/(2*(sigma^2)))*((RobotinoPos(1)-IRWerte(1,x))/(sigma^2));
    IRVY(x)=-K*exp(-((RobotinoPos(1)-IRWerte(1,x))^2+(RobotinoPos(2)-IRWerte(2,x))^2)/(2*(sigma^2)))*((RobotinoPos(2)-IRWerte(2,x))/(sigma^2));
       else
    IRVX=0;
    IRVY=0;
       end
    else
    IRVX(x)=0;
    IRVY(x)=0;
    end
end


 
K=0.4; %Steigung der schrägen
x=RobotinoPos(1);
y=RobotinoPos(2);
x_test=0;
y_test=0;
VektorX=0;
VektorY=0;
%% Einteilung des Vektorbereichs in verschidene Zonen
%%Einbahnstraßen hinter und neben den Stationen
 if (x >601) && (x<=5301) && (y>2501) && (y<=3201)
    Zone=4;
elseif (x >2751) && (x<=5501) && (y>3201)
    Zone=1;
elseif (x > 601) && (x<=2751) && (y>3201)
    Zone=2;
 elseif (x<=601) && (y>2001) && (AlteZone ~= 0)
     Zone=3;  
 elseif (x >5001) && (y>2501) && (AlteZone==1 || AlteZone==5)
     Zone=5;
 else
     Zone=0;
 end

KE=1000;
sigma=50;
Parabel=1000; 
 if Zone == 0 % Hauptfahrbereich
     if (x <= 5500) && (y <= 2500)
         x_test=(1/sigma)*KE*exp(-x/sigma);
         y_test=(-1/sigma)*KE*exp((y-2500)/sigma);
     elseif (x > 5500) && (y <= 2500)
         x_test=(1/sigma)*KE*exp((-(x-5500)+(y-2500))/sigma);
         y_test=(-1/sigma)*KE*exp((-(x-5500)+(y-2500))/sigma);
     elseif (x > 5500) && (y > 2500)
         x_test=(1/sigma)*KE*exp(-(x-5500)/sigma);
         y_test=(-1/sigma)*KE*exp((y-3600)/sigma);
     end
 MVX=x_test+(-1/sigma)*KE*exp((x-7400)/sigma);
 MVY=y_test+(1/sigma)*KE*exp(-y/sigma);
 
 VektorX=sum(SVX(5:6))+sum(RVX)+ZVX+sum(IRVX)-MVX;
 VektorY=sum(SVY(5:6))+sum(RVY)+ZVY+sum(IRVY)-MVY;
 elseif Zone == 1 %Rinne nach rechts weg
     ersterFifo=zeros([1 4]);
     for i=5:8
     ersterFifo(i)=floor((i-1)/2)*3+2*mod((i-1),2)+1;
     if sum(FifoArray(ersterFifo(i)))~=0
         MVX=0.25;
     else    
     MVX=K; 
     end
     end
     MVY=-2*(y-3500)/Parabel; % Parabel abgeleitet
 VektorX=sum(RVX)-MVX;
 VektorY=sum(RVY)-MVY;
 elseif Zone == 2 %Rinne nach links weg
     ersterFifo=zeros([1 4]);
     for i=1:4
     ersterFifo(i)=floor((i-1)/2)*3+2*mod((i-1),2)+1;
     if sum(FifoArray(ersterFifo(i)))~=0
         MVX=-0.25;
     else    
     MVX=-K; 
     end
     end
     MVY=-2*(y-3500)/Parabel; % Parabel abgeleitet
      VektorX=sum(RVX)-MVX;
      VektorY=sum(RVY)-MVY;
 elseif Zone == 3 %Rinne nach unten weg
     MVX=-2*(x-300)/Parabel; %Konstante Steigung
     MVY=-K; % Parabel abgeleitet
     VektorX=sum(RVX)+sum(IRVX)-MVX;
     VektorY=sum(RVY)+sum(IRVY)-MVY;
 elseif Zone == 5 %Rinne nach vorne weg aus Zone 1
     MVX=-2*(x-5500)/Parabel; %Konstante Steigung
     MVY=-K; % Parabel abgeleitet
     VektorX=sum(RVX)+sum(IRVX)-MVX;
     VektorY=sum(RVY)+sum(IRVY)-MVY;
 else % Bereich zwischen den Stationen
     MVX=0;
     MVY=K;
      VektorX=sum(RVX)+sum(SVX(1:4))-MVX;
      VektorY=sum(RVY)+sum(SVY(1:4))-MVY;
 end  
      Vektor(1)=VektorX;
      Vektor(2)=VektorY;
 end

== matlab function Gesamtmodell_Bahnplanung/Bahnplanung/Geschwindigkeit_begrenzen ==
  data: Vektor_In input; Vektor output; Transportbereich_aktiv input; RobPos input; IRDaten input; FilterIN input; Filter output
function [Vektor,Filter] = fcn(Vektor_In,Transportbereich_aktiv,RobPos,IRDaten,FilterIN)
Vektor=zeros([1 2]);
Filter=zeros([100 2]);
if (Transportbereich_aktiv==1) && (RobPos(1)>=0) && (RobPos(2)>=0)
    

 Filter(1,1)=Vektor_In(1);
 Filter(1,2)=Vektor_In(2);
 for x=1:99
     Filter(x+1,1)=FilterIN(x,1);
     Filter(x+1,2)=FilterIN(x,2);     
 end
 Vektor(1) =sum(Filter(:,1))/100;
 Vektor(2) =sum(Filter(:,2))/100;
 
 %Vektor(1) = Vektor_In(1);
 %Vektor(2) = Vektor_In(2);
 for x=1:9
if  (isnan(IRDaten(1,x))==0) && (IRDaten(1,x) <= 150)
    for x=1:2
    K=0.1; %Begrenzung langsame Zone
        if  Vektor(x)> K
            Vektor(x) = K;
        elseif Vektor(x) <-K
            Vektor(x)=-K;
        end
    end
end
 end
if (RobPos(2)<500)||(RobPos(2)>2300)
    for x=1:2
    K=0.3; %Begrenzung langsame Zone
        if  Vektor(x)> K
            Vektor(x) = K;
        elseif Vektor(x) <-K
            Vektor(x)=-K;
        end
    end
else
    for x=1:2
    K=0.7; %Begrenzung schnelle Zone
        if  Vektor(x)> K
            Vektor(x) = K;
        elseif Vektor(x) <-K
            Vektor(x)=-K;
        end
    end
end
end

== matlab function Gesamtmodell_Bahnplanung/Regelung1/Bereichswaehler ==
  data: modus output; transportbereich input; enable output; fertigungsbereich input
function [modus, enable] = fcn(transportbereich, fertigungsbereich)

enable = false;
modus = 0;

if fertigungsbereich == 1 && transportbereich == 0
    enable = true;
    modus = 1;
end
    
if fertigungsbereich == 0 && transportbereich == 1
    enable = true;
    modus = 0;
end

== matlab function Gesamtmodell_Bahnplanung/Regelung1/Kalman ==
  data: vxZustand input; vyZustand input; vPsiZustand input; PsiZustand input; xZustand input; yZustand input; enable input; dt parameter; vx output; vy output; vpsi output; pospsi output; posx output; posy output; enableBeob output
function [vx,vy,vpsi,pospsi,posx,posy,enableBeob] = fcn(vxZustand,vyZustand,vPsiZustand,PsiZustand,xZustand,yZustand,enable,dt)

persistent A H Q R 
persistent x P
persistent firstRun found
QVel = 0.01; 
QPos = 0.01;
if isempty(firstRun)
found = 0;
x = [0; 0; 0; 0; 2000; 1600];
    

A= [1       0       0       0       0       0;
    0       1       0       0       0       0;
    0       0       1       0       0       0;
    0       0       dt      1       0       0;
    dt      0       0       0       1       0;
    0       dt      0       0       0       1];
    
H = [0 0 0 1 0 0;
     0 0 0 0 1 0;
     0 0 0 0 0 1];

Q = [QVel       0       0       0       0       0;
     0       QVel       0       0       0       0;
     0          0       QVel    0       0       0;
     0          0       0       QPos    0       0;
     0          0       0       0       QPos    0;
     0          0       0       0       0    QPos];
   
  R = 1;

  P =  [1       0       0       0       0       0;
        0       1       0       0       0       0;
        0       0       1       0       0       0;
        0       0       0       1000       0       0;
        0       0       0       0       1000       0;
        0       0       0       0       0       1000];
  
  firstRun = 1;  
end


x =[vxZustand ; vyZustand; vPsiZustand;x(4:end,1)];

x = A*x;  
P = A*P*A' + Q;    
dist = 0;
Rnow = R;
if enable == 1
    z = [PsiZustand;xZustand;yZustand];
    % Reduzierung der Glaubwürdigkeit bei weit entfernten Messungen
    dist = sqrt(abs(z(2)-x(5))^2 + abs(z(3)-x(6))^2);

    
    if dist > 500
        Rnow = 0;
        found = 0;
    elseif dist > 100
        Rnow = 0;
        found = 0;
    elseif dist > 20
        Rnow = 0;
        found = 1;
    elseif dist < 20
        found =1;
        Rnow = 0;
    else 
        Rnow = R;
    end
    
    K =    P*H'*inv(H*P*H' + Rnow*eye(3)); 

    x = x + K*(z - H*x);

    P = P - K*H*P;
end
enableBeob = found;

vx      = x(1);
vy      = x(2);
vpsi    = x(3);
pospsi  = x(4);
posx    = x(5);
posy    = x(6);

== matlab function Gesamtmodell_Bahnplanung/Regelung1/NewCam ==
  data: yZustand input; xZustand input; psiZustand input; enable output
function enable = fcn(yZustand,xZustand,psiZustand)


persistent oldx oldy oldpsi firstRun

if isempty(firstRun)
   firstRun = 1;
   oldx     = -1;
   oldy     = -1;
   oldpsi   = -1;
   firstRun = 2;
end

if ( xZustand == 0 && yZustand == 0)
    firstRun = 1;
    enable = 0;
elseif firstRun < 2
    firstRun = firstRun +1;
    enable =0;
else  
    if((mod(firstRun,1) == 0)&&((oldx ~= xZustand) || (oldy ~= yZustand) || (oldpsi ~= psiZustand)))
        enable = 1;
       oldx     = xZustand;
       oldy     = yZustand;
       oldpsi   = psiZustand;

    else
        enable = 0;
    end
end

== matlab function Gesamtmodell_Bahnplanung/Regelung1/Receiver/UDP interface/stop signals ==
  data: rob_number input; udp_in input; enable_out output
%%%%%%%%%%%%%%%%%%%%%%%%%%%%%%%%%%%%%%%%%%%%%%%%%%%%%%%%%%%%%%%%%%%%%%%%%%%
% Leads the enable command through. The enable command turns the Robotino %
% inputs to selectable form.                                              %
%                                                                         %
% input: udp_in (vector of 56 elements containing the data sent by the    %
%                camera-model)                                            %
% outputs: enable_out (1 = inputs are in selectable form;                 %
%                      0 = inputs are set to 0)                           %
%          udp_out (vector of 56 elements containing the data sent by the %
%                   camera-model)                                         %
%%%%%%%%%%%%%%%%%%%%%%%%%%%%%%%%%%%%%%%%%%%%%%%%%%%%%%%%%%%%%%%%%%%%%%%%%%%
function enable_out  = fcn(rob_number, udp_in)
enable_out = [0, 0];
if (udp_in(rob_number * 3 - 2) <= 0) && ...
   (udp_in(rob_number * 3 - 1) <= 0) && (udp_in(rob_number * 3) <= 0)
    enable_out(1) = 0;
else
    enable_out(1) = 1;
end
enable_out(2) = udp_in(28);
